simulink model "MassSpringDamper"  (R2018b)
settings: Solver=VariableStepAuto  StartTime=0.0  StopTime=10.0  RelTol=1e-3
values from neighbouring files (symbols this model uses):
  x0 = 0.2    [parameters.m]
undefined symbols (not defined in the file or in its folder): c, k, k2, m
settings Model: Creator=Hannah  LastModifiedBy=Hannah

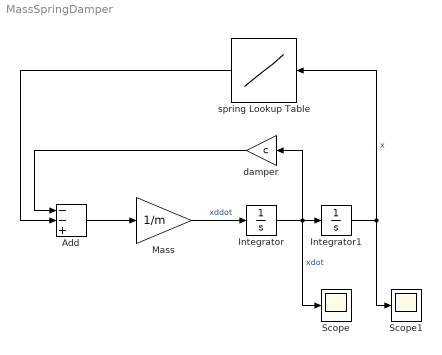
== system MassSpringDamper ==
  Add : Sum  Inputs=--+
  Integrator : Integrator
  Integrator1 : Integrator  InitialCondition=1
  "Mass " : Gain  Gain=1/m
  Scope : Scope
  Scope1 : Scope
  "damper " : Gain  Gain=c
  spring Lookup Table : Lookup_n-D  NumberOfTableDimensions=1  BreakpointsForDimension1=[-2*x0, -x0, x0, 2*x0]  Table=[-(k+k2)*x0, -k*x0, k*x0, (k+k2)*x0]  InternalRulePriority=Speed  RndMeth=Simplest  InputSameDT=on
  wires:
  "Mass "/1 -> Integrator/1  "xddot"
  Integrator/1 -> Scope/1, "damper "/1, Integrator1/1  "xdot"
  Integrator1/1 -> spring Lookup Table/1, Scope1/1  "x"
  spring Lookup Table/1 -> Add/2
  "damper "/1 -> Add/1
  Add/1 -> "Mass "/1
